simulink library "sm_boom_lift_crawler_lib_inputs"  (R2026a)
settings: Solver=VariableStepAuto
libraries: sm_boom_lift_crawler_lib x12
Description:
  | Boom Lift Crawler Motion Input Sequence
  | 
  | Copyright 2020-2026 The MathWorks, Inc.
settings Model: Creator=smiller  LastModifiedBy=smiller

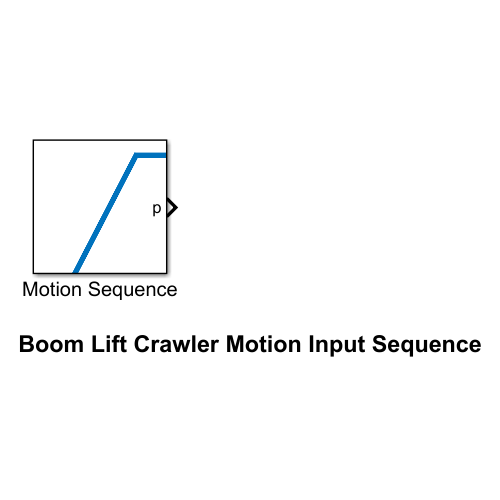
[thumbnail: Simulink's stored preview of the top-level diagram]
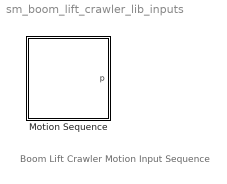
== system sm_boom_lift_crawler_lib_inputs ==
  note: Boom Lift Crawler Motion Input Sequence
  Motion Sequence : Subsystem
      mask Display: image('sm_boom_lift_crawler_motion_seq.svg');

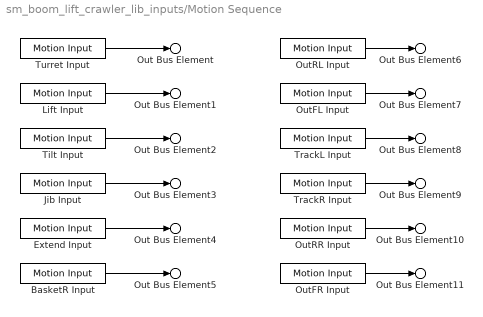
== system sm_boom_lift_crawler_lib_inputs/Motion Sequence ==
  BasketR Input : sm_boom_lift_crawler_lib/Motion Input  vec_t=motion.basketR.t  vec_q=motion.basketR.q
  Extend Input : sm_boom_lift_crawler_lib/Motion Input  vec_t=motion.extend.t  vec_q=motion.extend.p
  Jib Input : sm_boom_lift_crawler_lib/Motion Input  vec_t=motion.jib.t  vec_q=motion.jib.p
  Lift Input : sm_boom_lift_crawler_lib/Motion Input  vec_t=motion.lift.t  vec_q=motion.lift.p
  OutFL Input : sm_boom_lift_crawler_lib/Motion Input  vec_t=motion.outFL.t  vec_q=motion.outFL.p
  OutFR Input : sm_boom_lift_crawler_lib/Motion Input  vec_t=motion.outFR.t  vec_q=motion.outFR.p
  OutRL Input : sm_boom_lift_crawler_lib/Motion Input  vec_t=motion.outRL.t  vec_q=motion.outRL.p
  OutRR Input : sm_boom_lift_crawler_lib/Motion Input  vec_t=motion.outRR.t  vec_q=motion.outRR.p
  Tilt Input : sm_boom_lift_crawler_lib/Motion Input  vec_t=motion.tilt.t  vec_q=motion.tilt.p
  TrackL Input : sm_boom_lift_crawler_lib/Motion Input  vec_t=motion.TrackL.t  vec_q=motion.TrackL.p
  TrackR Input : sm_boom_lift_crawler_lib/Motion Input  vec_t=motion.TrackR.t  vec_q=motion.TrackR.p
  Turret Input : sm_boom_lift_crawler_lib/Motion Input  vec_t=motion.turret.t  vec_q=motion.turret.q
  Out Bus Element : Outport  PortName=p  Element=Turret
  Out Bus Element1 : Outport  PortName=p  Element=Lift
  Out Bus Element2 : Outport  PortName=p  Element=Tilt
  Out Bus Element3 : Outport  PortName=p  Element=Jib
  Out Bus Element4 : Outport  PortName=p  Element=Extend
  Out Bus Element5 : Outport  PortName=p  Element=BasketR
  Out Bus Element6 : Outport  PortName=p  Element=OutRL
  Out Bus Element7 : Outport  PortName=p  Element=OutFL
  Out Bus Element8 : Outport  PortName=p  Element=TrackL
  Out Bus Element9 : Outport  PortName=p  Element=TrackR
  Out Bus Element10 : Outport  PortName=p  Element=OutRR
  Out Bus Element11 : Outport  PortName=p  Element=OutFR
  wires:
  BasketR Input/1 -> Out Bus Element5/1
  OutFL Input/1 -> Out Bus Element7/1
  OutRL Input/1 -> Out Bus Element6/1
  TrackL Input/1 -> Out Bus Element8/1
  TrackR Input/1 -> Out Bus Element9/1
  Lift Input/1 -> Out Bus Element1/1
  Turret Input/1 -> Out Bus Element/1
  OutFR Input/1 -> Out Bus Element11/1
  Jib Input/1 -> Out Bus Element3/1
  OutRR Input/1 -> Out Bus Element10/1
  Extend Input/1 -> Out Bus Element4/1
  Tilt Input/1 -> Out Bus Element2/1
